simulink model "bonus"  (R2021b)
settings: Solver=VariableStepAuto  StartTime=0.0  StopTime=10.0  RelTol=1e-3
values from neighbouring files (symbols this model uses):
  A = [ 0 1 0; 12.077 -0.0014 0.1407; 0 0 -0.2606]    [Project_part_2_code.m]
  B = [0; -0.0281; 0.0519]    [Project_part_2_code.m]
  k = acker(A,B,p)    [Project_part_2_code.m]
  M = [1 1 0]    [Project_part_2_code.m]
  Y = Y'    [Project_part_2_code.m]
undefined symbols (not defined in the file or in its folder): E
settings Model: Creator=chand  LastModifiedBy=chand

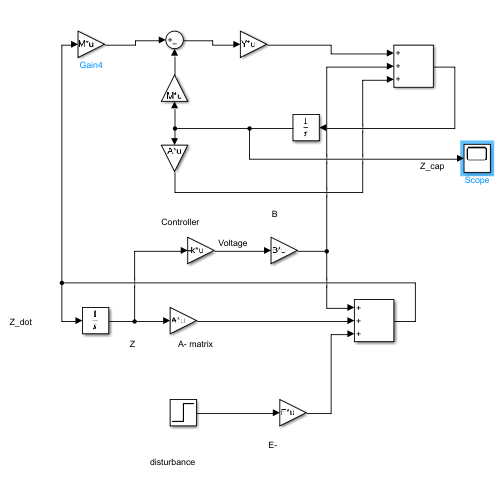
[thumbnail: Simulink's stored preview of the top-level diagram]
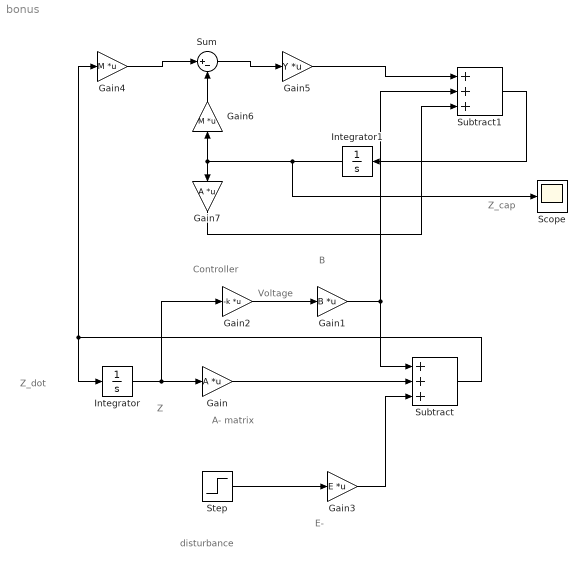
== system bonus ==
  note: disturbance
  note: E-
  note: A- matrix
  note: Z_dot
  note: Z
  note: B
  note: Controller
  note: Voltage
  note: Z_cap
  Gain : Gain  Gain=A  Multiplication=Matrix(K*u)
  Gain1 : Gain  Gain=B  Multiplication=Matrix(K*u)
  Gain2 : Gain  Gain=-k  Multiplication=Matrix(K*u)
  Gain3 : Gain  Gain=E  Multiplication=Matrix(K*u)
  Gain4 : Gain  Gain=M  Multiplication=Matrix(K*u)
  Gain5 : Gain  Gain=Y  Multiplication=Matrix(K*u)
  Gain6 : Gain  Gain=M  Multiplication=Matrix(K*u)
  Gain7 : Gain  Gain=A  Multiplication=Matrix(K*u)
  Integrator : Integrator
  Integrator1 : Integrator
  Scope : Scope
  Step : Step  SampleTime=0
  Subtract : Sum  Inputs=+++
  Subtract1 : Sum  Inputs=+++
  Sum : Sum  Inputs=|+-
  wires:
  Integrator/1 -> Gain2/1, Gain/1
  Gain1/1 -> Subtract/1, Subtract1/2
  Gain/1 -> Subtract/2
  Gain2/1 -> Gain1/1
  Step/1 -> Gain3/1
  Gain3/1 -> Subtract/3
  Subtract/1 -> Gain4/1, Integrator/1
  Gain4/1 -> Sum/1
  Gain6/1 -> Sum/2
  Sum/1 -> Gain5/1
  Gain5/1 -> Subtract1/1
  Integrator1/1 -> Scope/1, Gain7/1, Gain6/1
  Subtract1/1 -> Integrator1/1
  Gain7/1 -> Subtract1/3
